simulink model "DPT"  (R2023a)
settings: Solver=VariableStepAuto  StartTime=0.0  StopTime=0.1  RelTol=1e-3
libraries: simulink x2
settings Model: Creator=ПК  LastModifiedBy=ПК

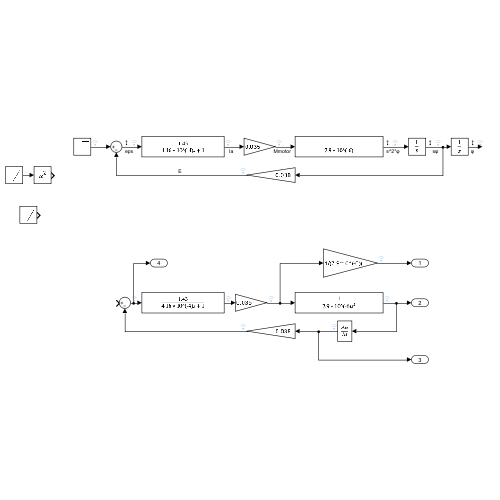
[thumbnail: Simulink's stored preview of the top-level diagram]
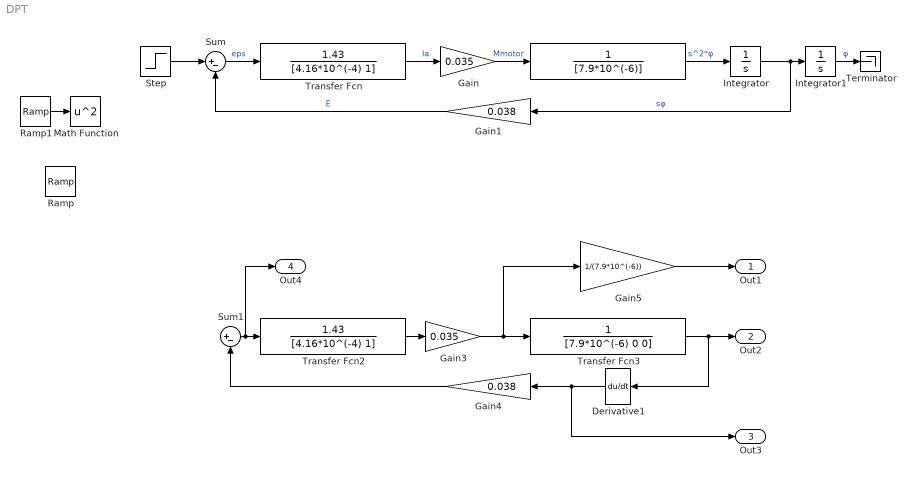
== system DPT ==
  " " : TransferFcn  Denominator=[7.9*10^(-6)]
  Derivative1 : Derivative  CoefficientInTFapproximation=10^(-4)
  Gain : Gain  Gain=0.035
  Gain1 : Gain  Gain=0.038
  Gain3 : Gain  Gain=0.035
  Gain4 : Gain  Gain=0.038
  Gain5 : Gain  Gain=1/(7.9*10^(-6))
  Integrator : Integrator
  Integrator1 : Integrator
  Math Function : Math  Operator=square
  Ramp : simulink/Sources/Ramp  slope=1000  start=0  InitialOutput=0
  Ramp1 : simulink/Sources/Ramp  slope=1000  start=0.01  InitialOutput=0
  Step : Step  Time=0  SampleTime=0
  Sum : Sum  Inputs=|+-
  Sum1 : Sum  Inputs=|+-
  Terminator : Terminator
  Transfer Fcn : TransferFcn  Numerator=[1.43]  Denominator=[4.16*10^(-4) 1]
  Transfer Fcn2 : TransferFcn  Numerator=[1.43]  Denominator=[4.16*10^(-4) 1]
  Transfer Fcn3 : TransferFcn  Denominator=[7.9*10^(-6) 0 0]
  Out1 : Outport
  Out2 : Outport  Port=2
  Out3 : Outport  Port=3
  Out4 : Outport  Port=4
  wires:
  Sum/1 -> Transfer Fcn/1  "eps"
  Transfer Fcn/1 -> Gain/1  "Ia"
  Gain/1 -> " "/1  "Mmotor"
  Gain1/1 -> Sum/2  "E"
  Gain4/1 -> Sum1/2
  Gain5/1 -> Out1/1
  Derivative1/1 -> Out3/1, Gain4/1
  Transfer Fcn3/1 -> Out2/1, Derivative1/1
  Sum1/1 -> Out4/1, Transfer Fcn2/1
  Gain3/1 -> Gain5/1, Transfer Fcn3/1
  Transfer Fcn2/1 -> Gain3/1
  Ramp1/1 -> Math Function/1
  " "/1 -> Integrator/1  "s^2*φ"
  Integrator/1 -> Integrator1/1, Gain1/1  "sφ"
  Integrator1/1 -> Terminator/1  "φ"
  Step/1 -> Sum/1
